simulink model "TwoTimeScale_Controller"  (R2023a)
settings: Solver=ode4  StartTime=0.0  StopTime=2  FixedStep=0.0005  RelTol=1e-3
settings Model: Creator=Fasih  LastModifiedBy=Fasih

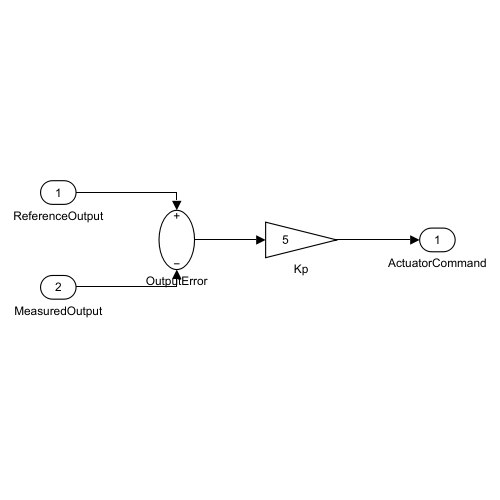
[thumbnail: Simulink's stored preview of the top-level diagram]
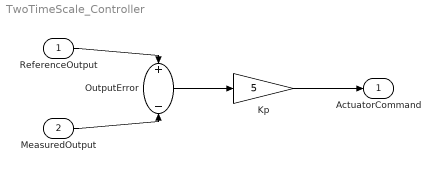
== system TwoTimeScale_Controller ==
  ReferenceOutput : Inport
  MeasuredOutput : Inport  Port=2
  Kp : Gain  Gain=5
  OutputError : Sum  Inputs=+-
  ActuatorCommand : Outport
  wires:
  ReferenceOutput/1 -> OutputError/1
  MeasuredOutput/1 -> OutputError/2
  OutputError/1 -> Kp/1
  Kp/1 -> ActuatorCommand/1
